simulink model "test_3ph_2w_transformer"  (R2018b)
settings: Solver=VariableStepAuto  StartTime=0.0  StopTime=10.0  RelTol=1e-3
undefined symbols (not defined in the file): S2
libraries: powerlib x12, typhoonHILlib x8
settings Model: Creator=USER  LastModifiedBy=USER

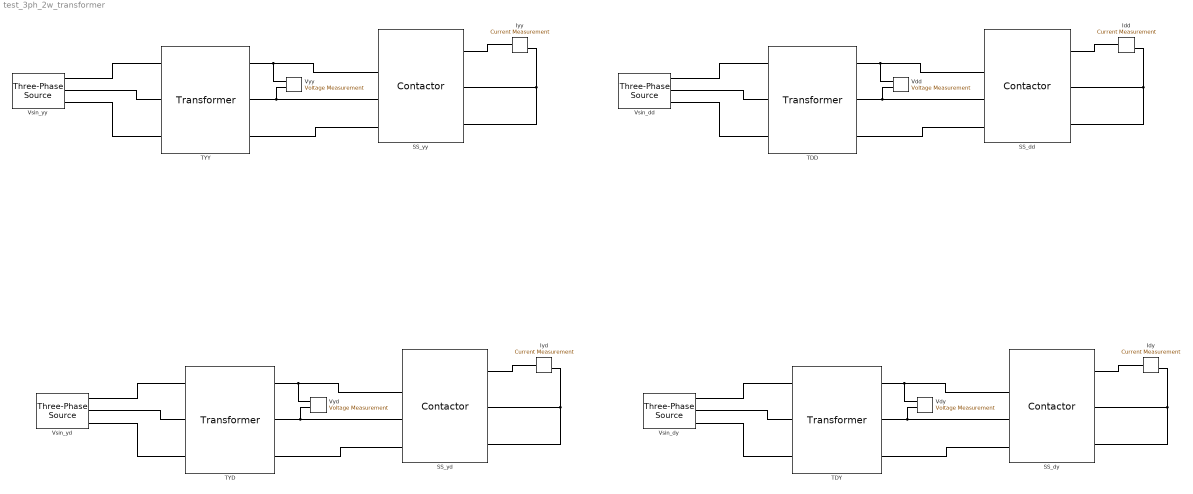
== system test_3ph_2w_transformer ==
  Idd : powerlib/Measurements/Current Measurement  PhasorSimulation=off  OutputType=Complex  PSBequivalent=0
  Idy : powerlib/Measurements/Current Measurement  PhasorSimulation=off  OutputType=Complex  PSBequivalent=0
  Iyd : powerlib/Measurements/Current Measurement  PhasorSimulation=off  OutputType=Complex  PSBequivalent=0
  Iyy : powerlib/Measurements/Current Measurement  PhasorSimulation=off  OutputType=Complex  PSBequivalent=0
  SS_dd : typhoonHILlib/Contactor  ContType=Triple Pole Single Throw  init_state=Off / S2  s1_logic=Active-high  di_1=1  tr1_delay=0  tr2_delay=0  r_on=0.001  v_f=0  r_s=1e4  c_s=inf  s0=0  toggle_init=on  old_pat=typhoonPatterns/TPST Contactor  old_size=140,185  model_loaded=off
      settings: SourceProductName=Typhoon HIL
  SS_dy : typhoonHILlib/Contactor  ContType=Triple Pole Single Throw  init_state=Off / S2  s1_logic=Active-high  di_1=1  tr1_delay=0  tr2_delay=0  r_on=0.001  v_f=0  r_s=1e4  c_s=inf  s0=0  toggle_init=on  old_pat=typhoonPatterns/TPST Contactor  old_size=140,185  model_loaded=off
      settings: SourceProductName=Typhoon HIL
  SS_yd : typhoonHILlib/Contactor  ContType=Triple Pole Single Throw  init_state=Off / S2  s1_logic=Active-high  di_1=1  tr1_delay=0  tr2_delay=0  r_on=0.001  v_f=0  r_s=1e4  c_s=inf  s0=0  toggle_init=on  old_pat=typhoonPatterns/TPST Contactor  old_size=140,185  model_loaded=off
      settings: SourceProductName=Typhoon HIL
  SS_yy : typhoonHILlib/Contactor  ContType=Triple Pole Single Throw  init_state=Off / S2  s1_logic=Active-high  di_1=1  tr1_delay=0  tr2_delay=0  r_on=0.001  v_f=0  r_s=1e4  c_s=inf  s0=0  toggle_init=on  old_pat=typhoonPatterns/TPST Contactor  old_size=140,185  model_loaded=off
      settings: SourceProductName=Typhoon HIL
  TDD : typhoonHILlib/Transformer  TransfType=Three-Phase Two Windings  Sn=10000  fn=50  Rm=1e5  Lm=100  sat_toggle=off  flux_vec=[0, 0.001, 0.005]  i_vec=[0, 1, 2]  n1=1  n2=1  coup12=off  coup13=off  coup14=off  units=SI  conn_1=Delta  V1=10000  R1=5  L1=1e-2  I1=0  conn_2=Delta  V2=400  R2=3  L2=5e-2  I2=0  conn_3=Wye  V3=100  R3=0.1  L3=1e-3  I3=0  conn_4=Wye  V4=100  R4=0.1  L4=1e-3  I4=0  toggle_init=on  old_pat=typhoonPatterns/TP 2W Transformer  old_size=145,176  model_loaded=off
      settings: SourceProductName=Typhoon HIL
  TDY : typhoonHILlib/Transformer  TransfType=Three-Phase Two Windings  Sn=10000  fn=50  Rm=1e7  Lm=100  sat_toggle=off  flux_vec=[0, 0.001, 0.005]  i_vec=[0, 1, 2]  n1=1  n2=1  coup12=off  coup13=off  coup14=off  units=SI  conn_1=Delta  V1=10000  R1=5  L1=1e-2  I1=0  conn_2=Wye  V2=400  R2=3  L2=5e-2  I2=0  conn_3=Wye  V3=100  R3=0.1  L3=1e-3  I3=0  conn_4=Wye  V4=100  R4=0.1  L4=1e-3  I4=0  toggle_init=on  old_pat=typhoonPatterns/TP 2W Transformer  old_size=145,176  model_loaded=off
      settings: SourceProductName=Typhoon HIL
  TYD : typhoonHILlib/Transformer  TransfType=Three-Phase Two Windings  Sn=10000  fn=50  Rm=1e5  Lm=100  sat_toggle=off  flux_vec=[0, 0.001, 0.005]  i_vec=[0, 1, 2]  n1=1  n2=1  coup12=off  coup13=off  coup14=off  units=SI  conn_1=Wye  V1=10000  R1=5  L1=1e-2  I1=0  conn_2=Delta  V2=400  R2=3  L2=5e-2  I2=0  conn_3=Wye  V3=100  R3=0.1  L3=1e-3  I3=0  conn_4=Wye  V4=100  R4=0.1  L4=1e-3  I4=0  toggle_init=on  old_pat=typhoonPatterns/TP 2W Transformer  old_size=145,176  model_loaded=off
      settings: SourceProductName=Typhoon HIL
  TYY : typhoonHILlib/Transformer  TransfType=Three-Phase Two Windings  Sn=10000  fn=50  Rm=1e5  Lm=100  sat_toggle=off  flux_vec=[0, 0.001, 0.005]  i_vec=[0, 1, 2]  n1=1  n2=1  coup12=off  coup13=off  coup14=off  units=SI  conn_1=Wye  V1=10000  R1=5  L1=1e-2  I1=0  conn_2=Wye  V2=400  R2=3  L2=5e-2  I2=0  conn_3=Wye  V3=100  R3=0.1  L3=1e-3  I3=0  conn_4=Wye  V4=100  R4=0.1  L4=1e-3  I4=0  toggle_init=on  old_pat=typhoonPatterns/TP 2W Transformer  old_size=145,176  model_loaded=off
      settings: SourceProductName=Typhoon HIL
  Vdd : powerlib/Measurements/Voltage Measurement  PhasorSimulation=off  OutputType=Complex  PSBequivalent=0
  Vdy : powerlib/Measurements/Voltage Measurement  PhasorSimulation=off  OutputType=Complex  PSBequivalent=0
  Vsin_dd : powerlib/Electrical Sources/Three-Phase Source  InternalConnection=Yg  VoltagePhases=off  Voltage=500  PhaseAngle=0  Voltage_phases=[25e3 25e3 25e3]/sqrt(3)  PhaseAngles_phases=[0 -120 +120]  Frequency=50  NonIdealSource=on  SpecifyImpedance=off  Resistance=0  Inductance=0  ShortCircuitLevel=100e6  BaseVoltage=0  XRratio=7  BusType=swing  Pref=10e3  Qref=0  Prefabc=[10e3, 10e3, 10e3]  Qrefabc=[0, 0, 0]  Qmin=-inf  Qmax=inf
  Vsin_dy : powerlib/Electrical Sources/Three-Phase Source  InternalConnection=Yg  VoltagePhases=off  Voltage=500  PhaseAngle=0  Voltage_phases=[25e3 25e3 25e3]/sqrt(3)  PhaseAngles_phases=[0 -120 +120]  Frequency=50  NonIdealSource=on  SpecifyImpedance=off  Resistance=0  Inductance=0  ShortCircuitLevel=100e6  BaseVoltage=0  XRratio=7  BusType=swing  Pref=10e3  Qref=0  Prefabc=[10e3, 10e3, 10e3]  Qrefabc=[0, 0, 0]  Qmin=-inf  Qmax=inf
  Vsin_yd : powerlib/Electrical Sources/Three-Phase Source  InternalConnection=Yg  VoltagePhases=off  Voltage=10000  PhaseAngle=0  Voltage_phases=[25e3 25e3 25e3]/sqrt(3)  PhaseAngles_phases=[0 -120 +120]  Frequency=50  NonIdealSource=on  SpecifyImpedance=off  Resistance=0  Inductance=0  ShortCircuitLevel=100e6  BaseVoltage=0  XRratio=7  BusType=swing  Pref=10e3  Qref=0  Prefabc=[10e3, 10e3, 10e3]  Qrefabc=[0, 0, 0]  Qmin=-inf  Qmax=inf
  Vsin_yy : powerlib/Electrical Sources/Three-Phase Source  InternalConnection=Yg  VoltagePhases=off  Voltage=500  PhaseAngle=0  Voltage_phases=[25e3 25e3 25e3]/sqrt(3)  PhaseAngles_phases=[0 -120 +120]  Frequency=50  NonIdealSource=on  SpecifyImpedance=off  Resistance=0  Inductance=0  ShortCircuitLevel=100e6  BaseVoltage=0  XRratio=7  BusType=swing  Pref=10e3  Qref=0  Prefabc=[10e3, 10e3, 10e3]  Qrefabc=[0, 0, 0]  Qmin=-inf  Qmax=inf
  "Vyd " : powerlib/Measurements/Voltage Measurement  PhasorSimulation=off  OutputType=Complex  PSBequivalent=0
  Vyy : powerlib/Measurements/Voltage Measurement  PhasorSimulation=off  OutputType=Complex  PSBequivalent=0
  connections:
  Vsin_yy/RConn1 -- TYY/LConn1
  TYY/LConn2 -- Vsin_yy/RConn2
  Vsin_yy/RConn3 -- TYY/LConn3
  SS_yy/LConn3 -- TYY/RConn3
  TYY/RConn2 -- Vyy/LConn2 -- SS_yy/LConn2
  SS_yy/LConn1 -- Vyy/LConn1 -- TYY/RConn1
  SS_yy/RConn1 -- Iyy/LConn1
  Iyy/RConn1 -- SS_yy/RConn2 -- SS_yy/RConn3
  TDD/RConn2 -- Vdd/LConn2 -- SS_dd/LConn2
  SS_dd/LConn1 -- Vdd/LConn1 -- TDD/RConn1
  Idd/RConn1 -- SS_dd/RConn2 -- SS_dd/RConn3
  TDD/LConn2 -- Vsin_dd/RConn2
  Vsin_dd/RConn3 -- TDD/LConn3
  SS_dd/LConn3 -- TDD/RConn3
  SS_dd/RConn1 -- Idd/LConn1
  Vsin_dd/RConn1 -- TDD/LConn1
  TYD/RConn2 -- "Vyd "/LConn2 -- SS_yd/LConn2
  Iyd/RConn1 -- SS_yd/RConn2 -- SS_yd/RConn3
  SS_yd/LConn1 -- "Vyd "/LConn1 -- TYD/RConn1
  Idy/RConn1 -- SS_dy/RConn2 -- SS_dy/RConn3
  SS_dy/LConn1 -- Vdy/LConn1 -- TDY/RConn1
  TDY/RConn2 -- Vdy/LConn2 -- SS_dy/LConn2
  Vsin_dy/RConn3 -- TDY/LConn3
  TYD/LConn2 -- Vsin_yd/RConn2
  SS_dy/RConn1 -- Idy/LConn1
  SS_yd/LConn3 -- TYD/RConn3
  Vsin_yd/RConn1 -- TYD/LConn1
  SS_yd/RConn1 -- Iyd/LConn1
  SS_dy/LConn3 -- TDY/RConn3
  Vsin_dy/RConn1 -- TDY/LConn1
  Vsin_yd/RConn3 -- TYD/LConn3
  TDY/LConn2 -- Vsin_dy/RConn2
